simulink model "SMC2"  (R2020b)
settings: Solver=VariableStepAuto  StartTime=0.0  StopTime=10.0  MaxStep=0.001  RelTol=1e-3
settings Model: Creator=MR.co  LastModifiedBy=Taha

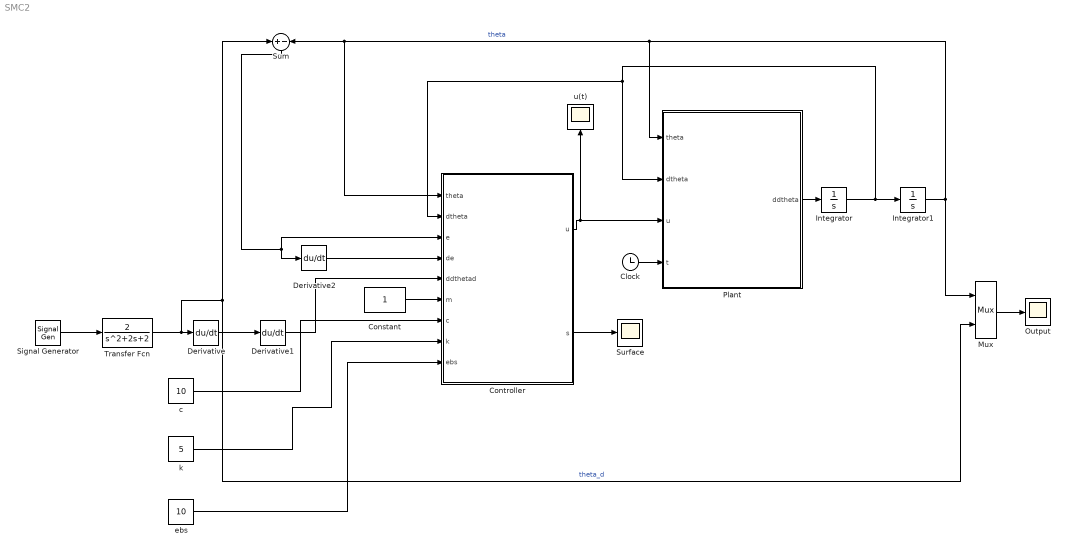
== system SMC2 ==
  Clock : Clock
  Constant : Constant
  Controller : MATLAB Function  TreatAsAtomicUnit=on
  Derivative : Derivative
  Derivative1 : Derivative
  Derivative2 : Derivative
  Integrator : Integrator  InitialCondition=randn
  Integrator1 : Integrator  InitialCondition=randn
  Mux : Mux  Inputs=2
  Output : Scope
  Plant : MATLAB Function  TreatAsAtomicUnit=on
  Signal Generator : SignalGenerator  Amplitude=10  Units=rad/sec
  Sum : Sum  Inputs=+|-
  Surface : Scope
  Transfer Fcn : TransferFcn  Numerator=[2]  Denominator=[1 2 2]
  c : Constant  Value=10
  ebs : Constant  Value=10
  k : Constant  Value=5
  u(t) : Scope
  wires:
  Controller/1(u) -> Plant/3(u), u(t)/1
  Plant/1(ddtheta) -> Integrator/1
  Integrator/1 -> Integrator1/1, Plant/2(dtheta), Controller/2(dtheta)
  Integrator1/1 -> Mux/1, Plant/1(theta), Controller/1(theta), Sum/2  "theta"
  Transfer Fcn/1 -> Mux/2, Sum/1, Derivative/1  "theta_d"
  Signal Generator/1 -> Transfer Fcn/1
  Derivative/1 -> Derivative1/1
  Derivative1/1 -> Controller/5(ddthetad)
  Sum/1 -> Derivative2/1, Controller/3(e)
  Derivative2/1 -> Controller/4(de)
  Mux/1 -> Output/1
  Clock/1 -> Plant/4(t)
  Controller/2(s) -> Surface/1
  Constant/1 -> Controller/6(m)
  c/1 -> Controller/7(c)
  k/1 -> Controller/8(k)
  ebs/1 -> Controller/9(ebs)

== matlab function SMC2/Controller ==
  data: theta input; dtheta input; e input; u output; de input; ddthetad input; s output; m input; c input; k input; ebs input
function [u , s]= fcn(theta , dtheta , e , de , ddthetad , m, c,k,ebs)
 %c = 10;
% ebs = 10;
% k = 5;
 s = de + c*e;

 delta = 0.001;

 dU = 10;
 dL = -10;
 d2 = (dU+dL)/2;
 d1 = (dU-dL)/2;
 dc = d2 - d1*sign(s);

    if m == 1
         u = 1/2 * (c * de + ebs*sign(s)  + ddthetad + k * s + theta + theta^3 + dtheta^2 -dc);
    elseif m == 2
         u = 1/2 * (c * de + ebs*tanh(s/delta)  + ddthetad + k * s + theta + theta^3 + dtheta^2 -dc);
    elseif m == 3
         u = 1/2 * (c * de + ebs*s/(abs(s)+delta)  + ddthetad + k * s + theta + theta^3 + dtheta^2 -dc);
    else
        if s>delta
             u = 1/2 * (c * de + ebs  + ddthetad + k * s + theta + theta^3 + dtheta^2 -dc);
        elseif s<-delta
             u = 1/2 * (c * de - ebs  + ddthetad + k * s + theta + theta^3 + dtheta^2 -dc);
        else
             u = 1/2 * (c * de + ebs*s/delta  + ddthetad + k * s + theta + theta^3 + dtheta^2 -dc);
        end
    end
end

== matlab function SMC2/Plant ==
  data: theta input; dtheta input; u input; ddtheta output; t input
function ddtheta = fcn(theta , dtheta , u ,t)

ddtheta = -theta - theta^3 - dtheta^2 + 2  *u + 10 * sin(pi*t);
